simulink model "canceladorEcoSimp"  (R2018a)
settings: Solver=VariableStepAuto  StartTime=0.0  StopTime=1500*Ts  RelTol=1e-3
InitFcn:
  | Ts = 1; %(s)
  | scramblerLocal = [3 5];
  | scramblerRemote = [5 7];
  | coefHybrid = [0 0.2 1 0.3 -0.4 -0.1 0.1 -0.05 -0.02 -0.01];
  | c_ik_init = [0 0 0 0 0];
  | mu = 0.02;
  | alpha = 0.9;
values from neighbouring files (symbols this model uses):
  G = 0.1    [lab3.m]
settings Model: Creator=leonardopedroso  LastModifiedBy=leonardopedroso

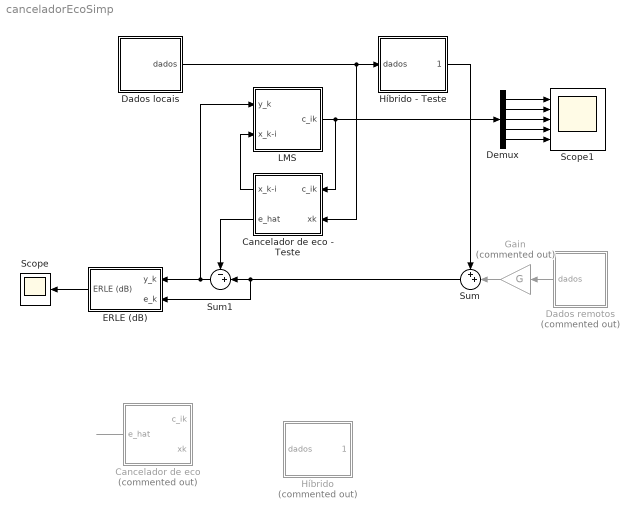
== system canceladorEcoSimp ==
  Cancelador de eco : Subsystem  Commented=on
  "Cancelador de eco - Teste " : Subsystem
  Dados locais : Subsystem
  Dados remotos : Subsystem  Commented=on
  Demux : Demux  Outputs=5
  ERLE (dB) : Subsystem
  Gain : Gain  Commented=on  Gain=G
  Híbrido : Subsystem  Commented=on
  Híbrido - Teste : Subsystem
  LMS : Subsystem
  Scope : Scope
  Scope1 : Scope  NumInputPorts=5
  Sum : Sum  Inputs=++|
  Sum1 : Sum  Inputs=-+|
  wires:
  Dados locais/1(dados) -> "Cancelador de eco - Teste "/2("xk "), Híbrido - Teste/1(dados)
  Híbrido - Teste/1(híbrido) -> Sum/1
  Gain/1 -> Sum/2
  Dados remotos/1(dados) -> Gain/1
  Sum/1 -> Sum1/2, ERLE (dB)/2(e_k)
  Cancelador de eco/1("e_hat ") -> ?
  LMS/1(c_ik) -> "Cancelador de eco - Teste "/1(c_ik), Demux/1
  Sum1/1 -> ERLE (dB)/1(y_k), LMS/1("y_k ")
  "Cancelador de eco - Teste "/2("e_hat ") -> Sum1/1
  "Cancelador de eco - Teste "/1(x_k-i) -> LMS/2(x_k-i)
  Demux/1 -> Scope1/1
  Demux/2 -> Scope1/2
  Demux/3 -> Scope1/3
  Demux/4 -> Scope1/4
  Demux/5 -> Scope1/5
  ERLE (dB)/1(ERLE (dB)) -> Scope/1

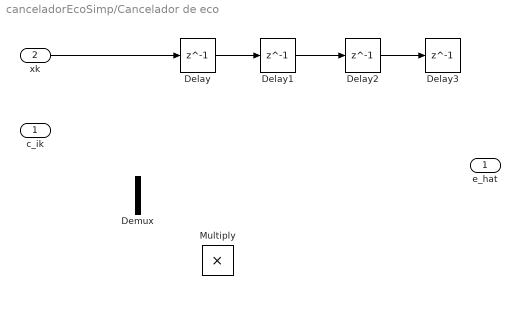
== system canceladorEcoSimp/Cancelador de eco ==
  c_ik : Inport
  "xk " : Inport  Port=2
  Delay{,1..3} (4 alike) : Delay  DelayLength=1  SampleTime=Ts
  Demux : Demux
  Multiply : Product
  "e_hat " : Outport
  wires:
  "xk "/1 -> Delay/1
  Delay/1 -> Delay1/1
  Delay1/1 -> Delay2/1
  Delay2/1 -> Delay3/1

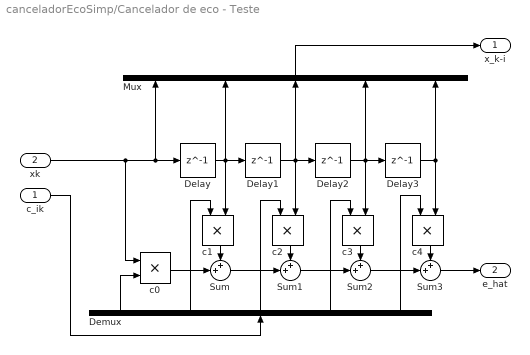
== system canceladorEcoSimp/Cancelador de eco - Teste  ==
  c_ik : Inport
  "xk " : Inport  Port=2
  Delay{,1..3} (4 alike) : Delay  DelayLength=1  SampleTime=Ts
  Demux : Demux  Outputs=5
  Mux : Mux  Inputs=5
  Sum{,1..3} (4 alike) : Sum  Inputs=++|
  c{0..4} (5 alike) : Product
  x_k-i : Outport
  "e_hat " : Outport  Port=2
  wires:
  "xk "/1 -> Delay/1, Mux/1, c0/1
  Delay/1 -> Delay1/1, Mux/2, c1/2
  Delay1/1 -> Mux/3, Delay2/1, c2/2
  Delay2/1 -> Mux/4, Delay3/1, c3/2
  Delay3/1 -> Mux/5, c4/2
  c1/1 -> Sum/1
  c0/1 -> Sum/2
  c3/1 -> Sum2/1
  c2/1 -> Sum1/1
  c4/1 -> Sum3/1
  Sum3/1 -> "e_hat "/1
  Sum/1 -> Sum1/2
  Sum1/1 -> Sum2/2
  Sum2/1 -> Sum3/2
  c_ik/1 -> Demux/1
  Demux/5 -> c4/1
  Demux/4 -> c3/1
  Demux/3 -> c2/1
  Demux/2 -> c1/1
  Demux/1 -> c0/2
  Mux/1 -> x_k-i/1

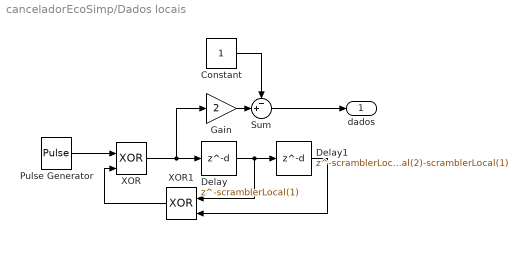
== system canceladorEcoSimp/Dados locais ==
  Constant : Constant
  Delay : Delay  DelayLength=scramblerLocal(1)  SampleTime=Ts
  Delay1 : Delay  DelayLength=scramblerLocal(2)-scramblerLocal(1)  SampleTime=Ts
  Gain : Gain  Gain=2
  Pulse Generator : DiscretePulseGenerator  PulseType=Time based  Period=2*Ts  PulseWidth=50
  Sum : Sum  Inputs=-+|
  XOR : Logic  Operator=XOR  IconShape=distinctive  AllPortsSameDT=off  OutDataTypeStr=boolean
  XOR1 : Logic  Operator=XOR  IconShape=distinctive  AllPortsSameDT=off  OutDataTypeStr=boolean
  dados : Outport
  wires:
  Pulse Generator/1 -> XOR/1
  XOR1/1 -> XOR/2
  Delay/1 -> XOR1/1, Delay1/1
  Delay1/1 -> XOR1/2
  Gain/1 -> Sum/2
  Constant/1 -> Sum/1
  XOR/1 -> Delay/1, Gain/1
  Sum/1 -> dados/1

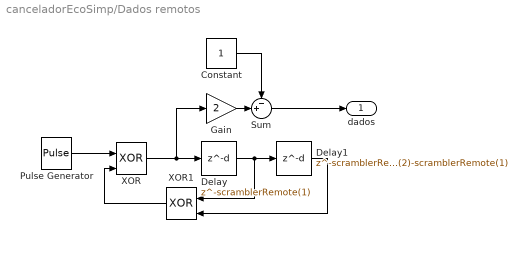
== system canceladorEcoSimp/Dados remotos ==
  Constant : Constant
  Delay : Delay  DelayLength=scramblerRemote(1)  SampleTime=Ts
  Delay1 : Delay  DelayLength=scramblerRemote(2)-scramblerRemote(1)  SampleTime=Ts
  Gain : Gain  Gain=2
  Pulse Generator : DiscretePulseGenerator  PulseType=Time based  Period=2*Ts  PulseWidth=50
  Sum : Sum  Inputs=-+|
  XOR : Logic  Operator=XOR  IconShape=distinctive  AllPortsSameDT=off  OutDataTypeStr=boolean
  XOR1 : Logic  Operator=XOR  IconShape=distinctive  AllPortsSameDT=off  OutDataTypeStr=boolean
  dados : Outport
  wires:
  Pulse Generator/1 -> XOR/1
  XOR1/1 -> XOR/2
  Delay/1 -> XOR1/1, Delay1/1
  Delay1/1 -> XOR1/2
  Gain/1 -> Sum/2
  Constant/1 -> Sum/1
  XOR/1 -> Delay/1, Gain/1
  Sum/1 -> dados/1

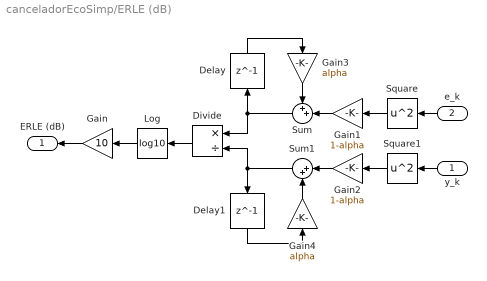
== system canceladorEcoSimp/ERLE (dB) ==
  y_k : Inport
  e_k : Inport  Port=2
  Delay : Delay  DelayLength=1  SampleTime=Ts
  Delay1 : Delay  DelayLength=1  SampleTime=Ts
  Divide : Product  Inputs=*/
  Gain : Gain  Gain=10
  Gain1 : Gain  Gain=1-alpha
  Gain2 : Gain  Gain=1-alpha
  Gain3 : Gain  Gain=alpha
  Gain4 : Gain  Gain=alpha
  Log : Math  Operator=log10  SaturateOnIntegerOverflow=on
  Square : Math  Operator=square  SaturateOnIntegerOverflow=on
  Square1 : Math  Operator=square  SaturateOnIntegerOverflow=on
  Sum : Sum  Inputs=++|
  Sum1 : Sum  Inputs=|++
  ERLE (dB) : Outport
  wires:
  Gain/1 -> ERLE (dB)/1
  Log/1 -> Gain/1
  Divide/1 -> Log/1
  e_k/1 -> Square/1
  y_k/1 -> Square1/1
  Square/1 -> Gain1/1
  Square1/1 -> Gain2/1
  Gain1/1 -> Sum/2
  Sum/1 -> Divide/1, Delay/1
  Delay/1 -> Gain3/1
  Gain3/1 -> Sum/1
  Delay1/1 -> Gain4/1
  Sum1/1 -> Divide/2, Delay1/1
  Gain2/1 -> Sum1/1
  Gain4/1 -> Sum1/2

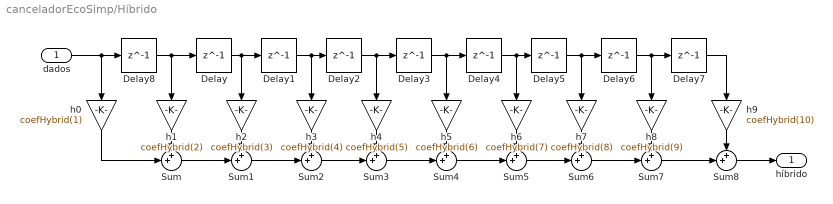
== system canceladorEcoSimp/Híbrido ==
  dados : Inport
  Delay{,1..8} (9 alike) : Delay  DelayLength=1  SampleTime=Ts
  Sum{,1..8} (9 alike) : Sum  Inputs=++|
  h0 : Gain  Gain=coefHybrid(1)
  h1 : Gain  Gain=coefHybrid(2)
  h2 : Gain  Gain=coefHybrid(3)
  h3 : Gain  Gain=coefHybrid(4)
  h4 : Gain  Gain=coefHybrid(5)
  h5 : Gain  Gain=coefHybrid(6)
  h6 : Gain  Gain=coefHybrid(7)
  h7 : Gain  Gain=coefHybrid(8)
  h8 : Gain  Gain=coefHybrid(9)
  h9 : Gain  Gain=coefHybrid(10)
  híbrido : Outport
  wires:
  dados/1 -> h0/1, Delay8/1
  Delay/1 -> h2/1, Delay1/1
  Delay1/1 -> h3/1, Delay2/1
  Delay2/1 -> Delay3/1, h4/1
  Delay3/1 -> h5/1, Delay4/1
  Delay4/1 -> h6/1, Delay5/1
  Delay6/1 -> Delay7/1, h8/1
  Delay5/1 -> Delay6/1, h7/1
  Delay7/1 -> h9/1
  h0/1 -> Sum/2
  Delay8/1 -> h1/1, Delay/1
  h1/1 -> Sum/1
  Sum8/1 -> híbrido/1
  Sum/1 -> Sum1/2
  h2/1 -> Sum1/1
  h3/1 -> Sum2/1
  Sum1/1 -> Sum2/2
  h4/1 -> Sum3/1
  Sum2/1 -> Sum3/2
  h5/1 -> Sum4/1
  Sum3/1 -> Sum4/2
  h6/1 -> Sum5/1
  Sum4/1 -> Sum5/2
  Sum5/1 -> Sum6/2
  h7/1 -> Sum6/1
  h8/1 -> Sum7/1
  h9/1 -> Sum8/1
  Sum7/1 -> Sum8/2
  Sum6/1 -> Sum7/2

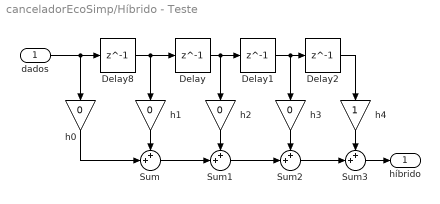
== system canceladorEcoSimp/Híbrido - Teste ==
  dados : Inport
  Delay{,1..2,8} (4 alike) : Delay  DelayLength=1  SampleTime=Ts
  Sum{,1..3} (4 alike) : Sum  Inputs=++|
  h{0..3} (4 alike) : Gain  Gain=0
  h4 : Gain
  híbrido : Outport
  wires:
  dados/1 -> h0/1, Delay8/1
  Delay/1 -> h2/1, Delay1/1
  Delay1/1 -> h3/1, Delay2/1
  Delay2/1 -> h4/1
  h0/1 -> Sum/2
  Delay8/1 -> h1/1, Delay/1
  h1/1 -> Sum/1
  Sum/1 -> Sum1/2
  h2/1 -> Sum1/1
  h3/1 -> Sum2/1
  Sum1/1 -> Sum2/2
  h4/1 -> Sum3/1
  Sum2/1 -> Sum3/2
  Sum3/1 -> híbrido/1

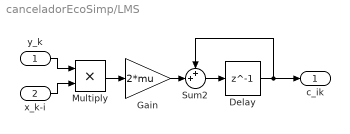
== system canceladorEcoSimp/LMS ==
  "y_k " : Inport
  x_k-i : Inport  Port=2
  Delay : Delay  DelayLength=1  InitialCondition=c_ik_init  SampleTime=Ts
  Gain : Gain  Gain=2*mu
  Multiply : Product
  Sum2 : Sum  Inputs=++|
  c_ik : Outport
  wires:
  Delay/1 -> c_ik/1, Sum2/1
  Gain/1 -> Sum2/2
  Sum2/1 -> Delay/1
  Multiply/1 -> Gain/1
  x_k-i/1 -> Multiply/2
  "y_k "/1 -> Multiply/1
